simulink model "MotorInteractionBench"  (R2024b)
settings: Solver=VariableStepAuto  StartTime=0.0  StopTime=50  RelTol=1e-3
model workspace (MATLAB code in the model file):
  | AllParams;
undefined symbols (not defined in the file): body
settings Model: Creator=Marij  LastModifiedBy=marijn
settings OptimizationCC: UseDivisionForNetSlopeComputation=on

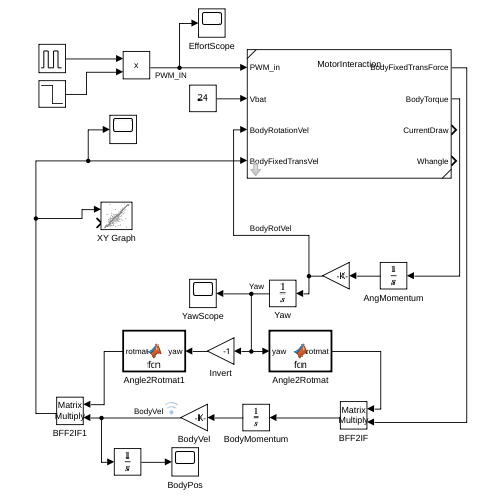
[thumbnail: Simulink's stored preview of the top-level diagram]
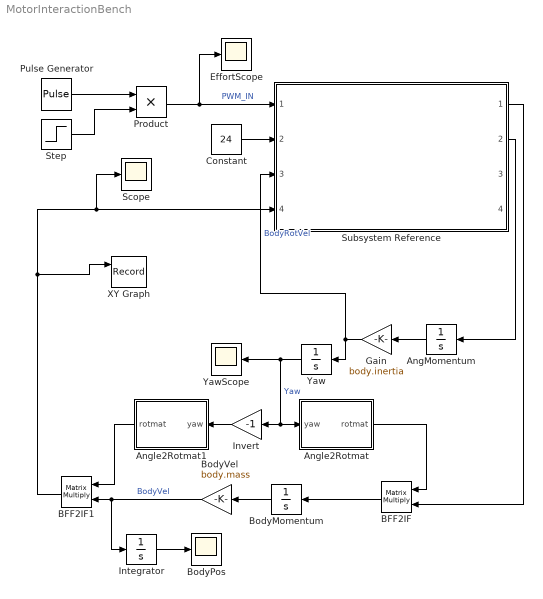
== system MotorInteractionBench ==
  AngMomentum : Integrator
  Angle2Rotmat : MATLAB Function  TreatAsAtomicUnit=on
  Angle2Rotmat1 : MATLAB Function  TreatAsAtomicUnit=on
  BFF2IF : Product  Multiplication=Matrix(*)
  BFF2IF1 : Product  Multiplication=Matrix(*)
  BodyMomentum : Integrator
  BodyPos : Scope
  BodyVel : Gain  Gain=body.mass
  Constant : Constant  Value=24
  EffortScope : Scope
  Gain : Gain  Gain=body.inertia
  Integrator : Integrator
  Invert : Gain  Gain=-1
  Product : Product
  Pulse Generator : DiscretePulseGenerator  PulseType=Time based  Amplitude=0.1  Period=5  PulseWidth=50  PhaseDelay=2.5
  Scope : Scope
  Step : Step  Time=5  Before=1  After=0  SampleTime=0
  Subsystem Reference : Subsystem  ReferencedSubsystem=MotorInteraction  whangle=1
  XY Graph : Record  FileSettingsInternal="{\"entries\":[{\"content\":{\"excelSettings\":{\"content\":{},\"type\":\"Streamout.ExcelSettings\"}},\"type\":\"Streamout.FileSettingStorage\",\"uuid\":\"\"}],\"packageUris\":[\"http:\\/\\/schema.mathworks.com\\/mf0\\/streamout_blocks\\/R2020a\"],\"version\":\"1.0\"}"  Layout=[1 1]  SignalsInternal="{\"entries\":[{\"content\":{\"signals\":[{\"content\":{\"blockPath\":[],\"dimensions\":[2],\"domain\":\"\",\"hasChildren\":true,\"lineColor\":\"#d95319\",\"lineWidth\":2,\"port\":1,\"signalID\":1,\"signalName\":\"BFF2IF1\"},\"type\":\"RecordBlkView.Signal\",\"uuid\":\"\"},{\"content\":{\"blockPath\":[],\"channel\":[1],\"dimensions\":[2],\"domain\":\"\",\"lineColor\":\"#4dbeee\",\"lineWidth\":2,\"parentID\":1,\"plots\":[ 1 ],\"port\":1,\"signalID\":2,\"signalName\":\"BFF2IF1\"},\"type\":\"RecordBlkView.Signal\",\"uuid\":\"\"},{\"content\":{\"blockPath\":[],\"channel\":[2],\"dimensions\":[2],\"domain\":\"\",\"lineColor\":\"#ff6929\",\"lineWidth\":2,\"parentID\":1,\"plots\":[ 1 ],\"port\":1,\"signalID\":3,\"signalName\":\"BFF2IF1\"},\"type\":\"RecordBlkView.Signal\",\"uuid\":\"\"},{\"content\":{\"blockPath\":[],\"dimensions\":[1],\"domain\":\"\",\"lineColor\":\"#0072bd\",\"lineWidth\":2,\"port\":2,\"signalID\":4},\"type\":\"RecordBlkView.Signal\",\"uuid\":\"\"}]},\"type\":\"RecordBlkView.InputSignals\",\"uuid\":\"\"}],\"packageUris\":[\"http:\\/\\/schema.mathworks.com\\/mf0\\/streamout_blocks\\/R2020a\"],\"version\":\"1.0\"}"  VisualizationBindings="{\"xyplotplugin\":{\"info\":[{\"series\":[{\"bindingParametersList\":[{\"parameter\":\"X-Axis\",\"signalID\":2,\"signalName\":\"BFF2IF1(1)\"},{\"parameter\":\"Y-Axis\",\"signalID\":3,\"signalName\":\"BFF2IF1(2)\"}],\"seriesID\":0}],\"subplotID\":1}]}}"  CompatibilityTag=XY
  Yaw : Integrator
  YawScope : Scope
  wires:
  Constant/1 -> Subsystem Reference/2
  Subsystem Reference/2 -> AngMomentum/1
  AngMomentum/1 -> Gain/1
  Gain/1 -> Subsystem Reference/3, Yaw/1  "BodyRotVel"
  Yaw/1 -> Invert/1, Angle2Rotmat/1(yaw), YawScope/1  "Yaw"
  Angle2Rotmat/1(rotmat) -> BFF2IF/1
  Subsystem Reference/1 -> BFF2IF/2
  BFF2IF/1 -> BodyMomentum/1
  BodyMomentum/1 -> BodyVel/1
  BodyVel/1 -> Integrator/1, BFF2IF1/2  "BodyVel"
  Invert/1 -> Angle2Rotmat1/1(yaw)
  Angle2Rotmat1/1(rotmat) -> BFF2IF1/1
  BFF2IF1/1 -> XY Graph/1, Scope/1, Subsystem Reference/4
  Pulse Generator/1 -> Product/1
  Product/1 -> EffortScope/1, Subsystem Reference/1  "PWM_IN"
  Step/1 -> Product/2
  Integrator/1 -> BodyPos/1

== matlab function MotorInteractionBench/Angle2Rotmat ==
  data: yaw input; rotmat output
function rotmat = fcn(yaw)
rotmat = [cos(yaw), -sin(yaw); sin(yaw), cos(yaw)];

== matlab function MotorInteractionBench/Angle2Rotmat1 ==
  data: yaw input; rotmat output
function rotmat = fcn(yaw)
rotmat = [cos(yaw), -sin(yaw); sin(yaw), cos(yaw)];
